simulink subsystem "Operator"  (R2022b)
settings: Solver=VariableStepAuto  StartTime=0.0  StopTime=10.0  RelTol=1e-3
settings Model: Creator=david  LastModifiedBy=david

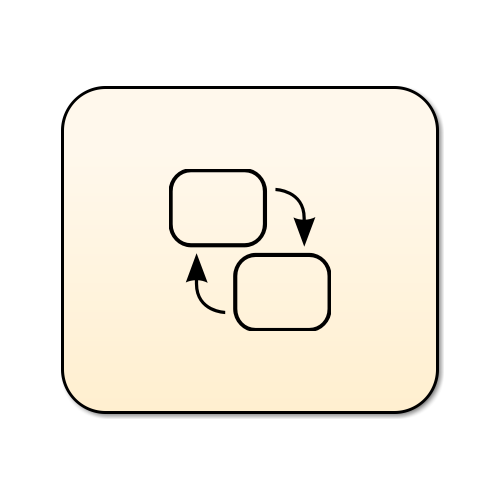
[thumbnail: Simulink's stored preview of the top-level diagram]
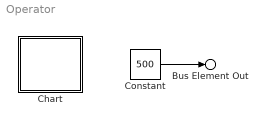
== system Operator ==
  Chart : Stateflow chart  TreatAsAtomicUnit=on
  Constant : Constant  Value=500
  Bus Element Out : Outport  VectorParamsAs1DForOutWhenUnconnected=off  PortName=Operator  Element=Trans.Speed_Command
  wires:
  Constant/1 -> Bus Element Out/1

== stateflow chart Operator/Chart ==
